simulink model "ground_state"  (R2017b)
settings: Solver=VariableStepAuto  StartTime=0.0  StopTime=10  RelTol=1e-3
undefined symbols (not defined in the file or in its folder): K
settings Model: Creator=benma  LastModifiedBy=benma

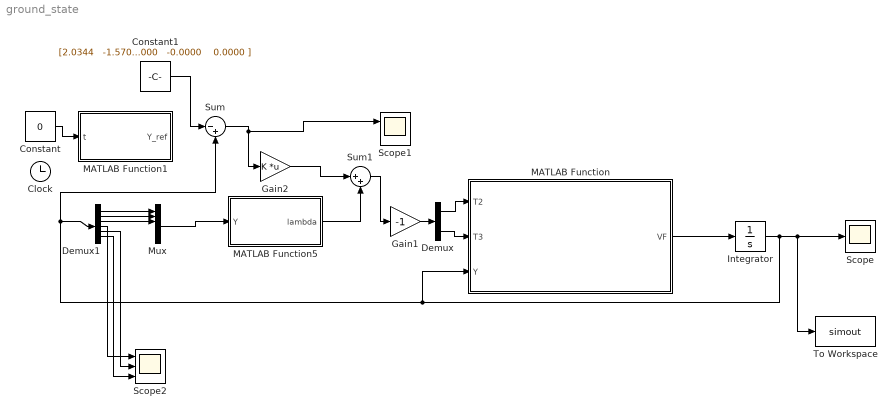
== system ground_state ==
  Clock : Clock
  Constant : Constant  Value=0
  Constant1 : Constant  Value=|
      | [2.0344   -1.5708    1.5708    0.0000   -0.0000    0.0000
      | ]
  Demux : Demux  Outputs=2
  Demux1 : Demux  Outputs=6
  Gain1 : Gain  Gain=-1
  Gain2 : Gain  Gain=K  Multiplication=Matrix(K*u)
  Integrator : Integrator  InitialCondition=|
      | [ 2.0344   -1.5708    1.5708    0.0000   -0.0000    0.0000
      | ]
  MATLAB Function : MATLAB Function  TreatAsAtomicUnit=on
  MATLAB Function1 : MATLAB Function  TreatAsAtomicUnit=on
  MATLAB Function5 : MATLAB Function  TreatAsAtomicUnit=on
  Mux : Mux  Inputs=6
  Scope : Scope
  Scope1 : Scope  NumInputPorts=2
  Scope2 : Scope  NumInputPorts=3
  Sum : Sum  Inputs=|-+
  Sum1 : Sum  Inputs=|++
  To Workspace : ToWorkspace  VariableName=simout  SaveFormat=Timeseries  SampleTime=-1
  wires:
  Integrator/1 -> To Workspace/1, Scope/1, MATLAB Function/3(Y), Demux1/1, Sum/2
  MATLAB Function/1(VF) -> Integrator/1
  Gain1/1 -> Demux/1
  Demux/1 -> MATLAB Function/1(T2)
  Demux/2 -> MATLAB Function/2(T3)
  Sum1/1 -> Gain1/1
  Sum/1 -> Scope1/1, Gain2/1
  Constant/1 -> MATLAB Function1/1(t)
  Gain2/1 -> Sum1/1
  Constant1/1 -> Sum/1
  MATLAB Function5/1(lambda) -> Sum1/2
  Demux1/1 -> Mux/1
  Demux1/6 -> Scope2/3
  Demux1/5 -> Scope2/2
  Demux1/4 -> Scope2/1
  Demux1/3 -> Mux/3
  Demux1/2 -> Mux/2
  Mux/1 -> MATLAB Function5/1(Y)

== matlab function ground_state/MATLAB Function ==
  data: T2 input; VF output; T3 input; Y input
function VF = threedof_ground(T2,T3,Y)
%THREEDOF_GROUND
%    VF = THREEDOF_GROUND(T2,T3,Y)

%    This function was generated by the Symbolic Math Toolbox version 8.0.
%    23-Nov-2018 17:29:58

t2 = Y(2);
t3 = t2.*2.0;
t4 = Y(3);
t5 = t4.*2.0;
t6 = Y(1);
t7 = Y(4);
t8 = t7.^2;
t9 = t2-t4;
t10 = sin(t9);
t11 = Y(5);
t12 = Y(6);
t13 = t2+t5;
t14 = sin(t13);
t15 = t11.^2;
t16 = cos(t5);
t17 = cos(t13);
t18 = t3+t5;
t19 = sin(t2);
t20 = t2+t4;
t21 = sin(t20);
t22 = t12.^2;
t23 = cos(t2);
t24 = cos(t3);
t25 = t24.*8.1e1;
t26 = t16.*4.5e1;
t27 = cos(t18);
t66 = t27.*9.0;
t28 = t25+t26-t66-1.69e2;
t29 = 1.0./t28;
t30 = cos(t6);
t31 = t3+t6;
t32 = cos(t31);
t33 = t32.*1.32435e4;
t34 = -t5+t6;
t35 = cos(t34);
t36 = t35.*4.4145e3;
t37 = t5+t6;
t38 = cos(t37);
t39 = t38.*4.4145e3;
t40 = t3+t5+t6;
t41 = cos(t40);
t42 = sin(t3);
t43 = sin(t5);
t44 = t8.*t10.*4.5e2;
t45 = t10.*t15.*4.5e2;
t46 = t10.*t22.*4.5e2;
t47 = t3+t4;
t48 = sin(t47);
t49 = cos(t9);
t50 = T3.*t17.*9.0e2;
t51 = sin(t18);
t52 = t15.*t19.*2.25e3;
t53 = sin(t4);
t54 = t8.*t21.*2.5e2;
t55 = t15.*t21.*2.5e2;
t56 = t21.*t22.*2.5e2;
t57 = cos(t20);
t58 = T3.*t57.*2.1e3;
t59 = t7.*t11.*t21.*5.0e2;
t60 = t7.*t12.*t21.*5.0e2;
t61 = t11.*t12.*t21.*5.0e2;
t62 = t7.*t10.*t11.*9.0e2;
t63 = t7.*t10.*t12.*9.0e2;
t64 = t10.*t11.*t12.*9.0e2;
t65 = t7.*t11.*t19.*4.5e3;
t67 = t2+t6;
t68 = cos(t67);
t69 = t68.*2.20725e4;
t70 = t2+t5+t6;
t71 = cos(t70);
t72 = -t2+t6;
t73 = cos(t72);
t74 = t2+t5-t6;
t75 = cos(t74);
t76 = t75.*4.4145e3;
t77 = t8.*t42.*1.35e3;
t78 = t15.*t42.*1.35e3;
t79 = t22.*t48.*4.5e2;
t80 = cos(t47);
t81 = T3.*t27.*9.0e2;
t82 = T2.*t23.*2.7e3;
t83 = cos(t4);
t84 = t7.*t11.*t42.*2.7e3;
t85 = t7.*t12.*t48.*9.0e2;
t86 = t11.*t12.*t48.*9.0e2;
VF = [t7;t11;t12;t29.*(T2.*2.3e3-t30.*3.1392e4+t33+t36+t39-t41.*1.4715e3+t44+t45+t46+t50+t52+t54+t55+t56+t58+t59+t60+t61+t62+t63+t64+t65+t77+t82-T2.*t16.*9.0e2-T2.*t17.*9.0e2-T3.*t23.*2.7e3-T3.*t49.*2.7e3-t8.*t14.*1.5e2+t8.*t19.*2.25e3-t14.*t15.*1.5e2-t8.*t51.*1.5e2-t7.*t11.*t14.*3.0e2).*(-3.0./5.0e1);t29.*(T2.*7.0e3-T3.*4.7e3-t30.*3.1392e4+t33+t36+t39-t41.*1.4715e3+t44+t45+t46+t50+t52+t54+t55+t56+t58+t59+t60+t61+t62+t63+t64+t65+t69-t71.*2.943e3-t73.*2.6487e4+t76+t78+t79+t81+t84+t85+t86-T2.*t16.*9.0e2-T2.*t17.*1.8e3+T2.*t23.*5.4e3-T3.*t23.*2.7e3-T2.*t27.*9.0e2-T3.*t49.*2.7e3+T3.*t80.*2.7e3-T3.*t83.*5.7e3-t8.*t14.*9.0e2+t8.*t19.*7.2e3-t14.*t15.*1.5e2+t8.*t42.*2.7e3-t8.*t43.*7.5e2+t8.*t48.*4.5e2-t15.*t43.*7.5e2-t8.*t51.*1.5e2-t8.*t53.*1.45e3+t15.*t48.*4.5e2-t15.*t53.*1.45e3-t22.*t53.*1.45e3-t7.*t11.*t14.*3.0e2-t7.*t11.*t43.*1.5e3+t7.*t11.*t48.*9.0e2-t7.*t11.*t53.*2.9e3-t7.*t12.*t53.*2.9e3-t11.*t12.*t53.*2.9e3).*(3.0./5.0e1);t29.*(T2.*4.7e3-T3.*1.9e4+t69-t71.*2.943e3-t73.*2.6487e4+t76+t77+t78+t79+t81+t82+t84+t85+t86-cos(t2+t4+t6).*2.4525e3+cos(t2+t4-t6).*5.886e3+cos(t2-t4+t6).*8.829e3-cos(-t2+t4+t6).*1.32435e4-T2.*t17.*9.0e2+T3.*t24.*8.1e3-T2.*t27.*9.0e2+T2.*t49.*2.7e3-T2.*t57.*2.1e3-T2.*t80.*2.7e3+T3.*t80.*5.4e3+T2.*t83.*5.7e3-T3.*t83.*1.14e4+t8.*t10.*2.25e3-t8.*t14.*7.5e2+t8.*t19.*4.95e3-t8.*t21.*8.5e2-t8.*t43.*1.5e3+t8.*t48.*9.0e2-t15.*t43.*1.5e3+t8.*t51.*1.5e2-t8.*t53.*5.0e3+t15.*t48.*9.0e2-t22.*t43.*7.5e2+t15.*t51.*1.5e2-t15.*t53.*5.0e3+t22.*t51.*1.5e2-t22.*t53.*1.45e3-t7.*t11.*t43.*3.0e3-t7.*t12.*t43.*1.5e3+t7.*t11.*t48.*1.8e3-t11.*t12.*t43.*1.5e3+t7.*t11.*t51.*3.0e2+t7.*t12.*t51.*3.0e2-t7.*t11.*t53.*1.0e4-t7.*t12.*t53.*2.9e3+t11.*t12.*t51.*3.0e2-t11.*t12.*t53.*2.9e3).*(-3.0./5.0e1)];

== matlab function ground_state/MATLAB Function1 ==
  data: t input; Y_ref output
function Y_ref = Refrence(t)
%REFRENCE
%    Y_REF = REFRENCE(T)

%    This function was generated by the Symbolic Math Toolbox version 8.0.
%    25-Nov-2018 00:13:09

t2 = t.^2;
t3 = exp(t2);
t4 = 1.0./sqrt(t3);
t5 = t.*5.0;
t6 = exp(t5);
t7 = exp(-2.5e1./2.0);
t8 = t4.*t6.*t7.*(2.0./5.0);
t9 = cos(t8);
t10 = sin(t8);
t11 = t-5.0;
t12 = t11.^2;
t26 = t12.*(1.0./2.0);
t13 = exp(-t26);
t14 = t9.^2;
t15 = t10.^2;
t23 = t10.*4.0;
t16 = t14+t15-t23+4.0;
t17 = sqrt(t16);
t18 = t9+t17;
t19 = t10-2.0;
t20 = 1.0./t19;
t21 = t4.*t6.*t7.*2.0;
t24 = t.*t4.*t6.*t7.*(2.0./5.0);
t22 = t21-t24;
t25 = 1.0./t19.^2;
t27 = t11.*t13.*(2.0./5.0);
Y_ref = [atan(t18.*t20).*-2.0;t13.*(-2.0./5.0)-pi.*(1.0./2.0);t13.*(2.0./5.0)+pi.*(1.0./2.0);(t20.*(t10.*t22+t9.*1.0./sqrt(t16).*t22.*2.0).*2.0+t9.*t18.*t22.*t25.*2.0)./(t18.^2.*t25+1.0);t27;-t27];

== matlab function ground_state/MATLAB Function5 ==
  data: Y input; lambda output
function lambda = ridgid_torque(Y)
%RIDGID_TORQUE
%    LAMBDA = RIDGID_TORQUE(Y)

%    This function was generated by the Symbolic Math Toolbox version 8.0.
%    24-Nov-2018 22:24:49

t2 = Y(2);
t3 = Y(3);
t4 = Y(1);
t5 = t2.*2.0;
t6 = Y(4);
t7 = sin(t5);
t8 = Y(5);
t9 = t6.^2;
t10 = t2-t3;
t11 = sin(t10);
t12 = t8.^2;
t13 = t3.*2.0;
t14 = Y(6);
t15 = t3+t5;
t16 = sin(t15);
t17 = t2+t13;
t18 = sin(t17);
t19 = t14.^2;
t20 = t5+t13;
t21 = sin(t20);
t22 = sin(t2);
t23 = t2+t3;
t24 = sin(t23);
t25 = sin(t3);
t26 = cos(t2);
t27 = t26.*3.0;
t28 = cos(t3);
t29 = cos(t23);
t30 = t27+t28+t29+4.0;
t31 = 1.0./t30;
t32 = cos(t4);
t33 = t2+t4;
t34 = cos(t33);
t35 = t3+t4;
t36 = cos(t35);
t37 = t2+t3-t4;
t38 = cos(t37);
t39 = t3+t4+t5;
t40 = cos(t39);
t41 = -t3+t4;
t42 = cos(t41);
t43 = t4+t5+t13;
t44 = cos(t43);
t45 = t44.*1.4715e3;
t46 = t2+t3+t4;
t47 = cos(t46);
t48 = sin(t13);
t49 = t9.*t11.*9.0e2;
t50 = t9.*t21.*3.0e2;
t51 = t12.*t21.*1.5e2;
t52 = t19.*t21.*1.5e2;
t53 = t9.*t24.*3.3e3;
t54 = t6.*t8.*t21.*3.0e2;
t55 = t6.*t14.*t21.*3.0e2;
t56 = t8.*t14.*t21.*3.0e2;
lambda = [t31.*(t32.*-3.4335e4+t34.*1.91295e4-t36.*1.03005e4-t38.*7.3575e3+t40.*8.829e3-t42.*1.03005e4+t45+t47.*6.3765e3+t49+t50+t51+t52+t53+t54+t55+t56-cos(-t2+t4).*2.20725e4+cos(t4+t5).*1.32435e4+t7.*t9.*2.7e3+t7.*t12.*1.35e3+t11.*t12.*9.0e2+t9.*t16.*1.8e3+t9.*t18.*3.0e2+t12.*t16.*9.0e2+t11.*t19.*4.5e2+t12.*t18.*3.0e2+t9.*t22.*7.5e3+t12.*t22.*3.3e3+t16.*t19.*4.5e2+t12.*t24.*1.9e3+t18.*t19.*1.5e2+t19.*t22.*4.5e2+t19.*t24.*5.5e2-t19.*t25.*9.5e2+t6.*t7.*t8.*2.7e3+t6.*t8.*t11.*1.8e3+t6.*t8.*t16.*1.8e3+t6.*t11.*t14.*9.0e2+t6.*t8.*t18.*6.0e2+t8.*t11.*t14.*9.0e2+t6.*t8.*t22.*6.6e3+t6.*t14.*t16.*9.0e2+t6.*t8.*t24.*3.8e3+t6.*t14.*t18.*3.0e2+t8.*t14.*t16.*9.0e2+t8.*t14.*t18.*3.0e2+t6.*t14.*t22.*9.0e2+t6.*t14.*t24.*1.1e3+t8.*t14.*t22.*9.0e2-t6.*t14.*t25.*1.9e3+t8.*t14.*t24.*1.1e3-t8.*t14.*t25.*1.9e3).*8.333333333333333e-4;t31.*(t32.*(-8.3385e3)-t34.*4.4145e3+t36.*1.4715e3-t38.*7.3575e3+t40.*4.4145e3-t42.*1.1772e4+t45+t47.*9.81e3-t49+t50+t51+t52+t53+t54+t55+t56+cos(t2+t4+t13).*1.4715e3-cos(t2-t3+t4).*4.4145e3-t11.*t12.*4.5e2+t9.*t16.*9.0e2+t9.*t18.*6.0e2+t12.*t16.*4.5e2+t12.*t18.*4.5e2+t9.*t25.*3.3e3+t12.*t22.*4.5e2+t12.*t24.*1.55e3+t12.*t25.*1.95e3+t18.*t19.*3.0e2+t19.*t24.*2.0e2+t19.*t25.*2.0e2+t9.*t48.*3.0e2+t12.*t48.*3.0e2+t19.*t48.*1.5e2-t6.*t8.*t11.*9.0e2+t6.*t8.*t16.*9.0e2+t6.*t8.*t18.*9.0e2+t6.*t8.*t22.*9.0e2+t6.*t8.*t24.*3.1e3+t6.*t14.*t18.*6.0e2+t6.*t8.*t25.*3.9e3+t8.*t14.*t18.*6.0e2+t6.*t14.*t24.*4.0e2+t6.*t14.*t25.*4.0e2+t8.*t14.*t24.*4.0e2+t8.*t14.*t25.*4.0e2+t6.*t8.*t48.*6.0e2+t6.*t14.*t48.*3.0e2+t8.*t14.*t48.*3.0e2).*8.333333333333333e-4];
